simulink model "saturn_ib_stack_test"  (Simulink 6.2)
settings: Solver=ode4  SolverMode=SingleTasking  StartTime=-20.0  StopTime=620  FixedStep=0.005  RelTol=1e-3
values from neighbouring files (symbols this model uses):
  A_z_deg = 82.8200    (= 82.82)    [AS205_presettings.m]
  BN_1_sec = 14.4    [AS205_presettings.m]
  DeltaV_b_mps = 7.2381    [AS205_presettings.m]
  epsilon_2_sec = 15.0    (= 15)    [AS205_presettings.m]
  epsilon_prime_sec = 3.0    (= 3)    [AS205_presettings.m]
  i_deg = 28.89597    [AS205_presettings.m]
  lambda_0_deg = 102.32900    (= 102.329)    [AS205_presettings.m]
  lambda_L_deg = -80.561141    [AS205_presettings.m]
  pad_roll_L_deg = 100.0    (= 100)    [AS205_presettings.m]
  phi_L_deg = 28.521963    [AS205_presettings.m]
  phi_L_prime_deg = 28.360795    [AS205_presettings.m]
  R_L_m = 6373385.0    (= 6373385)    [AS205_presettings.m]
  R_T_m = 6570774.0    (= 6570774)    [AS205_presettings.m]
  T3_FM_sec = 6.08    [AS205_presettings.m]
  T_HSL_sec = 5.0    (= 5)    [AS205_presettings.m]
  Theta_T_deg = 0.000    (= 0)    [AS205_presettings.m]
  V_T_mps = 7780.976    [AS205_presettings.m]
  Xdotdot_VGT_mps2 = -9.251    [AS205_presettings.m]
undefined symbols (not defined in the file or in its folder): e0_0, e1_0, e2_0, e3_0, m, s
libraries: simulink x99, aerolibconvert x83, aerolibutil x63, aerolibtransform2 x34, aerolibasang x2, aerolibatmos2 x2, aerolib6dofsys x2
(part 1 of 7)
CloseFcn:
  | rtwprivate ssgencode ModelCloseRequest Saturn_IB_CSM_test
settings Model: LastModifiedBy=riley  StrictBusMsg=ErrorLevel1
settings OptimizationCC: InlineParams=on  InlineInvariantSignals=on  EnforceIntegerDowncast=off
settings DebuggingCC: ArrayBoundsChecking=error  SignalInfNanChecking=error  AlgebraicLoopMsg=error  SolverPrmCheckMsg=warning  IntegerOverflowMsg=error  SFcnCompatibilityMsg=error
settings RTWCC: SystemTargetFile=grt_malloc.tlc  GenCodeOnly=on  TemplateMakefile=grt_malloc_default_tmf  Description=Generic Real-Time Target with dynamic memory allocation  ProcessScript=grt_malloc_make_rtw_hook
settings GRTTargetCC: UtilityFuncGeneration=Shared location

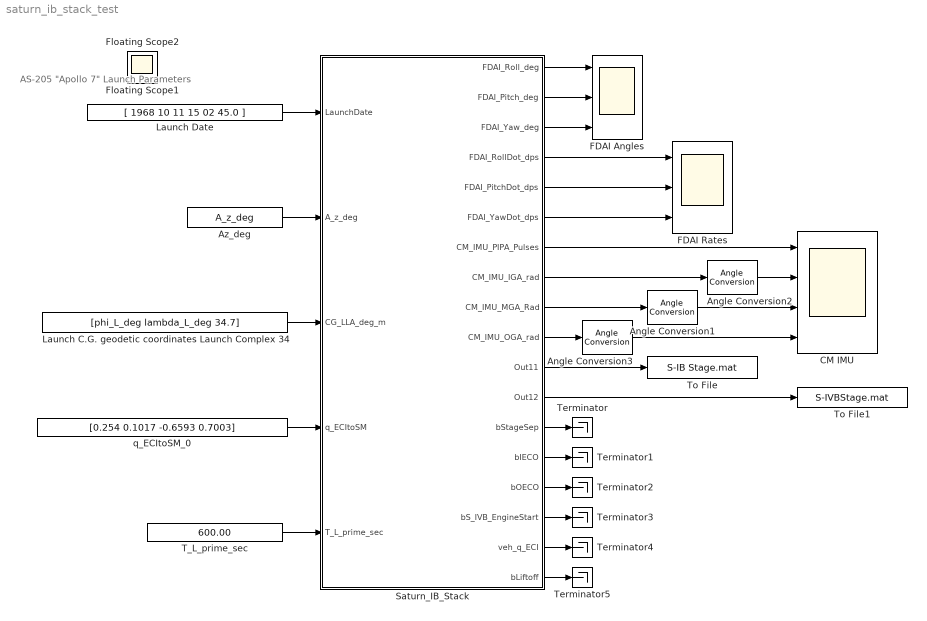
== system saturn_ib_stack_test ==
  note: AS-205 "Apollo 7" Launch Parameters
  Angle Conversion1 : aerolibconvert/Angle Conversion  IU=rad  OU=deg
  Angle Conversion2 : aerolibconvert/Angle Conversion  IU=rad  OU=deg
  Angle Conversion3 : aerolibconvert/Angle Conversion  IU=rad  OU=deg
  Az_deg : Constant  Value=A_z_deg
  CM IMU : Scope  NumInputPorts=4
      settings: YMin=-3500~90.002~-0.005~-17.188  YMax=500~90.015~0.035~-17.179  SaveName=ScopeData11
  FDAI Angles : Scope  NumInputPorts=3
      settings: YMin=-18~85.5~-0.02  YMax=0~90.25~0.06  SaveName=ScopeData8
  FDAI Rates : Scope  NumInputPorts=3
      settings: YMin=-0.07~-0.35~-0.05  YMax=0.005~-5.55112e-017~0.04  SaveName=ScopeData7
  Launch C.G. geodetic coordinates Launch Complex 34 : Constant  Value=[phi_L_deg lambda_L_deg 34.7]
  Launch Date : Constant  Value=[ 1968 10 11 15 02 45.0 ]
  Saturn_IB_Stack : Subsystem
  T_L_prime_sec : Constant  Value=600.00
  Terminator{,1..5} (6 alike) : Terminator
  To File : ToFile  Filename=S-IB Stage.mat  SampleTime=0.04
  To File1 : ToFile  Filename=S-IVBStage.mat  MatrixName=ans_sivb  SampleTime=0.04
  q_ECItoSM_0 : Constant  Value=[0.254 0.1017 -0.6593 0.7003]
  Floating Scope1 : Scope
      settings: Floating=on  SaveName=ScopeData16
  Floating Scope2 : Scope
      settings: Floating=on  SaveName=ScopeData17
  wires:
  Az_deg/1 -> Saturn_IB_Stack/2(A_z_deg)
  Launch Date/1 -> Saturn_IB_Stack/1(LaunchDate)
  Launch C.G. geodetic coordinates Launch Complex 34/1 -> Saturn_IB_Stack/3(CG_LLA_deg_m)
  Saturn_IB_Stack/4(FDAI_RollDot_dps) -> FDAI Rates/1
  Saturn_IB_Stack/7(CM_IMU_PIPA_Pulses) -> CM IMU/1
  Saturn_IB_Stack/10(CM_IMU_OGA_rad) -> Angle Conversion3/1
  Angle Conversion2/1 -> CM IMU/2
  Angle Conversion1/1 -> CM IMU/3
  Angle Conversion3/1 -> CM IMU/4
  Saturn_IB_Stack/1(FDAI_Roll_deg) -> FDAI Angles/1
  Saturn_IB_Stack/2(FDAI_Pitch_deg) -> FDAI Angles/2
  Saturn_IB_Stack/3(FDAI_Yaw_deg) -> FDAI Angles/3
  Saturn_IB_Stack/5(FDAI_PitchDot_dps) -> FDAI Rates/2
  Saturn_IB_Stack/6(FDAI_YawDot_dps) -> FDAI Rates/3
  Saturn_IB_Stack/8(CM_IMU_IGA_rad) -> Angle Conversion2/1
  Saturn_IB_Stack/9(CM_IMU_MGA_Rad) -> Angle Conversion1/1
  Saturn_IB_Stack/11(Out11) -> To File/1
  Saturn_IB_Stack/12(Out12) -> To File1/1
  Saturn_IB_Stack/13(bStageSep) -> Terminator/1
  Saturn_IB_Stack/14(bIECO) -> Terminator1/1
  Saturn_IB_Stack/15(bOECO) -> Terminator2/1
  Saturn_IB_Stack/16(bS_IVB_EngineStart) -> Terminator3/1
  q_ECItoSM_0/1 -> Saturn_IB_Stack/4(q_ECItoSM)
  Saturn_IB_Stack/17(veh_q_ECI) -> Terminator4/1
  Saturn_IB_Stack/18(bLiftoff) -> Terminator5/1
  T_L_prime_sec/1 -> Saturn_IB_Stack/5(T_L_prime_sec)

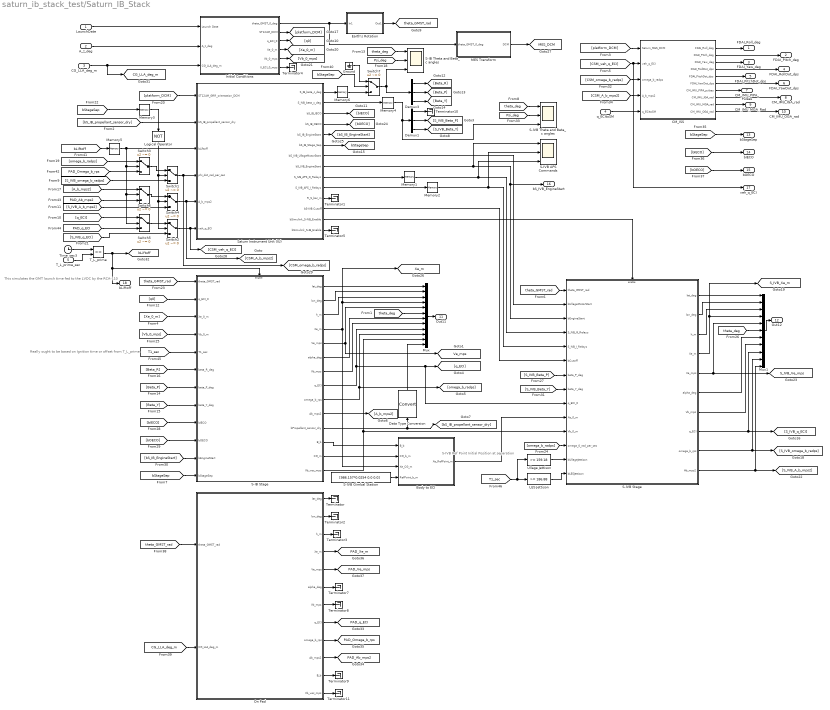
== system saturn_ib_stack_test/Saturn_IB_Stack ==
  note: S-IVB Ref Point Initial
      | Position at separation
  note: Really ought to be based on
      | Ignition time or offset
      | from T_L_prime
  note: This simulates the
      | GMT launch time
      | fed to the LVDC by
      | the RCA-110
  LaunchDate : Inport  Port=1  PortDimensions=6  DataType=double  LatchInput=off
  A_z_deg : Inport  Port=2  PortDimensions=1  DataType=double  LatchInput=off
  CG_LLA_deg_m : Inport  Port=3  PortDimensions=3  DataType=double  LatchInput=off
  q_ECItoSM : Inport  Port=4  PortDimensions=4  DataType=double  LatchInput=off
  T_L_prime_sec : Inport  Port=5  PortDimensions=1  DataType=double  LatchInput=off
  Body to ECI : Subsystem
  CM_ISS : Subsystem
  Data Type Conversion : DataTypeConversion  Orientation=up
  Demux1 : Demux  Outputs=3
  Demux3 : Demux  Outputs=3
  Earth's Rotation : Subsystem
  Ground : Ground
  Initial Conditions : Subsystem
  LES Jettison : simulink/Logic and Bit Operations/Compare To Constant  relop=>=  const=186.88  LogicOutDataTypeMode=boolean  ZeroCross=off
  Logical Operator : Logic  Orientation=down  Operator=NOT  AllPortsSameDT=off  OutDataTypeMode=Boolean
  MES Transform : Subsystem
  Memory{1..6} (6 alike) : Memory  InheritSampleTime=on
  Mux : Mux  Inputs=12
  Mux1 : Mux  Inputs=11
  On Pad : Subsystem
  S-IB Stage : Subsystem
  S-IB Theta and Beta_c angles : Scope  NumInputPorts=3
      settings: YMin=-18~-1.3~-0.04  YMax=1~0.3~0.14  SaveName=ScopeData2  Decimation=10  SampleTime=0.01
  S-IVB APS Commands : Scope  NumInputPorts=3
      settings: TimeRange=620  YMin=0.95~-1~-1  YMax=1.05~1~1  SaveName=ScopeData3  MaxDataPoints=15000  Decimation=10  SampleTime=0.01
  S-IVB Gimbal Station : Constant  Value=[986.157*0.0254 0.0 0.0]
  S-IVB Stage : Subsystem
  S-IVB Theta and Beta_c angles : Scope  NumInputPorts=3
      settings: YMin=-65~-0.075~-0.5  YMax=5~0.425~0.8  SaveName=ScopeData12  MaxDataPoints=15000  Decimation=10  SampleTime=0.01
  Saturn Instrument Unit (IU) : Subsystem
  Switch{1..7} (7 alike) : Switch  Criteria=u2 ~= 0
  T_L_prime : RelationalOperator  LogicOutDataTypeMode=Boolean
  Terminator{,1..5,7..11} (11 alike) : Terminator
  Time_sec3 : Clock
  Ullage Jettison : simulink/Logic and Bit Operations/Compare To Constant  relop=>=  const=159.18  LogicOutDataTypeMode=boolean  ZeroCross=off
  FDAI_Roll_deg : Outport  PortDimensions=1
  FDAI_Pitch_deg : Outport  Port=2  PortDimensions=1
  FDAI_Yaw_deg : Outport  Port=3  PortDimensions=1
  FDAI_RollDot_dps : Outport  Port=4
  FDAI_PitchDot_dps : Outport  Port=5
  FDAI_YawDot_dps : Outport  Port=6
  CM_IMU_PIPA_Pulses : Outport  Port=7
  CM_IMU_IGA_rad : Outport  Port=8
  CM_IMU_MGA_Rad : Outport  Port=9
  CM_IMU_OGA_rad : Outport  Port=10
  Out11 : Outport  Port=11
  Out12 : Outport  Port=12
  bStageSep : Outport  Port=13  DataType=boolean
  bIECO : Outport  Port=14  DataType=boolean
  bOECO : Outport  Port=15  DataType=boolean
  bS_IVB_EngineStart : Outport  Port=16  DataType=boolean
  veh_q_ECI : Outport  Port=17  PortDimensions=4  DataType=double
  bLiftoff : Outport  Port=18  DataType=boolean
  tag scope: CG_LLA_deg_m=global, MES_DCM=global, PAD_Ab_mps2=global, PAD_Omega_b_rps=global, PAD_Ve_mps=global, PAD_Xe_m=global, PAD_q_ECI=global, S_IVB_Ve_mps=global, S_IVB_Xe_m=global, Ve_mps=global, Xe_m=global, bLiftoff=global, bStageSep=global, theta_GMST_rad=global
  wires:
  Earth's Rotation/1(Out1) -> [theta_GMST_rad]
  Initial Conditions/1(theta_GMST_0_deg) -> Earth's Rotation/1(In1), MES Transform/1(theta_GMST_0_deg)
  Initial Conditions/3(q_ECI_0) -> [q0]
  Initial Conditions/2(ST124M_DCM) -> [platform_DCM]
  [q0] -> S-IB Stage/2(q_ECI_0)
  [theta_GMST_rad] -> S-IB Stage/1(theta_GMST_rad)
  Initial Conditions/4(Xe_0_m) -> [Xe_0_m]
  [Xe_0_m] -> S-IB Stage/3(Xe_0_m)
  [Beta_Y] -> S-IB Stage/8(beta_Y_deg)
  Initial Conditions/5(Vb_0_mps) -> [Vb_0_mps]
  [Vb_0_mps] -> S-IB Stage/4(Vb_0_m)
  [Beta_R] -> S-IB Stage/6(beta_R_deg)
  [Beta_P] -> S-IB Stage/7(beta_P_deg)
  Demux3/3 -> [Beta_Y]
  Demux3/1 -> [Beta_R]
  Demux3/2 -> [Beta_P]
  [Psi_deg] -> S-IB Theta and Beta_c angles/2
  [theta_deg] -> S-IB Theta and Beta_c angles/1
  [platform_DCM] -> Saturn Instrument Unit (IU)/1(ST124M_GRR_orientation_DCM)
  [bS_IB_EngineStart] -> S-IB Stage/11(bEngineStart)
  [bOECO] -> S-IB Stage/10(bOECO)
  [bIECO] -> S-IB Stage/9(bIECO)
  S-IB Stage/4(Xe_m) -> Body to ECI/3(Xe_CG_m), Mux/4, [Xe_m]
  S-IB Stage/5(Ve_mps) -> [Ve_mps], Mux/5
  Saturn Instrument Unit (IU)/3(bS_IB_IECO) -> [bIECO]
  Saturn Instrument Unit (IU)/4(bS_IB_OECO) -> [bOECO]
  Saturn Instrument Unit (IU)/5(bS_IB_EngineStart) -> [bS_IB_EngineStart]
  S-IB Stage/1(lat_deg) -> Mux/1
  S-IB Stage/2(lon_deg) -> Mux/2
  S-IB Stage/3(h_m) -> Mux/3
  S-IB Stage/6(alpha_deg) -> Mux/7
  S-IB Stage/7(Vb_mps) -> Mux/8
  [theta_deg] -> Mux/6
  S-IB Stage/8(q_ECI) -> Mux/9, [q_ECI], S-IVB Stage/9(q_ECI_0)
  S-IB Stage/9(omega_b_rps) -> [omega_b_radps], Mux/10
  S-IB Stage/10(Ab_mps2) -> [A_b_mps2]
  [bS_IB_propellant_sensor_dry] -> Saturn Instrument Unit (IU)/2(bS_IB_propellant_sensor_dry)
  S-IB Stage/12(B_b) -> Body to ECI/1(B_b)
  S-IB Stage/13(CG_m) -> Body to ECI/2(CG_b_m)
  S-IVB Gimbal Station/1 -> Body to ECI/4(RefPoint_b_m)
  [bStageSep] -> S-IB Stage/12(bStageSep)
  Demux1/3 -> [S_IVB_Beta_Y]
  Demux1/1 -> Terminator10/1
  Demux1/2 -> [S_IVB_Beta_P]
  Saturn Instrument Unit (IU)/2(S_IVB_beta_c_deg) -> Memory4/1
  Switch2/1 -> Saturn Instrument Unit (IU)/6(veh_q_ECI), [CSM_veh_q_ECI]
  [S_IVB_omega_b_radps] -> Switch1/3
  [S_IVB_A_b_mps2] -> Switch4/3
  [S_IVB_q_ECI] -> Switch2/3
  [bStageSep] -> Memory3/1
  Logical Operator/1 -> Switch2/2, Switch4/2, Switch1/2
  S-IB Stage/14(Vb_vec_mps) -> Mux/11, S-IVB Stage/11(Vb_0_m)
  Data Type Conversion/1 -> Mux/12
  Initial Conditions/6(V_ECI_0_mps) -> Terminator4/1
  Saturn Instrument Unit (IU)/7(bS_IVB_UllageMotorStart) -> S-IVB Stage/2(bUllageMotorStart)
  Saturn Instrument Unit (IU)/8(bS_IVB_EngineStart) -> S-IVB APS Commands/1, S-IVB Stage/3(bEngineStart), bS_IVB_EngineStart/1
  Saturn Instrument Unit (IU)/9(S_IVB_APS_III_Relays) -> Memory1/1
  Saturn Instrument Unit (IU)/10(S_IVB_APS_I_Relays) -> Memory2/1
  Saturn Instrument Unit (IU)/13(bSimulink_S-IVB_Enable) -> S-IVB Stage/Enable
  S-IB Stage/11(bPropellant_sensor_dry) -> [bS_IB_propellant_sensor_dry], Data Type Conversion/1
  Saturn Instrument Unit (IU)/14(bSimulink_S-IB_Enable) -> Terminator5/1
  Switch1/1 -> [CSM_omega_b_radps], Saturn Instrument Unit (IU)/4(phi_dot_rad_per_sec)
  Switch4/1 -> Saturn Instrument Unit (IU)/5(A_b_mps2), [CSM_A_b_mps2]
  Saturn Instrument Unit (IU)/6(bS_IB_Stage_Sep) -> [bStageSep]
  S-IVB Stage/1(lat_deg) -> Mux1/1
  S-IVB Stage/6(alpha_deg) -> Mux1/7
  S-IVB Stage/5(Ve_mps) -> [S_IVB_Ve_mps], Mux1/5
  S-IVB Stage/2(lon_deg) -> Mux1/2
  [theta_GMST_rad] -> S-IVB Stage/1(theta_GMST_rad)
  Saturn Instrument Unit (IU)/12(bS-IVB Cutoff) -> S-IVB Stage/6(bCutoff)
  [S_IVB_Beta_P] -> S-IVB Stage/7(beta_P_deg)
  [S_IVB_Beta_Y] -> S-IVB Stage/8(beta_Y_deg)
  Body to ECI/1(Xe_RefPoint_m) -> S-IVB Stage/10(Xe_0_m)
  S-IVB Stage/8(q_ECI) -> [S_IVB_q_ECI], Mux1/9
  S-IVB Stage/9(omega_b_rps) -> [S_IVB_omega_b_radps], Mux1/10
  S-IVB Stage/10(Ab_mps2) -> [S_IVB_A_b_mps2], Mux1/11
  S-IVB Stage/7(Vb_mps) -> Mux1/8
  [theta_deg] -> Mux1/6
  S-IVB Stage/3(h_m) -> Mux1/3
  S-IVB Stage/4(Xe_m) -> Mux1/4, [S_IVB_Xe_m]
  [omega_b_radps] -> S-IVB Stage/12(omega_0_rad_per_sec)
  Memory1/1 -> S-IVB Stage/4(S_IVB_III_Relays), S-IVB APS Commands/3
  Memory3/1 -> Logical Operator/1
  [theta_deg] -> S-IVB Theta and Beta_c angles/1
  [Psi_deg] -> S-IVB Theta and Beta_c angles/2
  Ullage Jettison/1 -> S-IVB Stage/13(bUllageJettison)
  LES Jettison/1 -> S-IVB Stage/14(bLESJettison)
  MES Transform/1(DCM) -> [MES_DCM]
  Memory2/1 -> S-IVB Stage/5(S_IVB_I_Relays), S-IVB APS Commands/2
  Memory4/1 -> Demux1/1, S-IVB Theta and Beta_c angles/3
  Saturn Instrument Unit (IU)/11(R_S_bar_m) -> Terminator1/1
  [platform_DCM] -> CM_ISS/1(Saturn_MES_DCM)
  [CSM_veh_q_ECI] -> CM_ISS/2(veh_q_ECI), veh_q_ECI/1
  [CSM_omega_b_radps] -> CM_ISS/3(omega_b_radps)
  [CSM_A_b_mps2] -> CM_ISS/4(A_b_mps2)
  LaunchDate/1 -> Initial Conditions/1(Launch Date)
  A_z_deg/1 -> Initial Conditions/2(A_z_deg)
  CM_ISS/1(FDAI_Roll_deg) -> FDAI_Roll_deg/1
  CM_ISS/2(FDAI_Pitch_deg) -> FDAI_Pitch_deg/1
  CM_ISS/3(FDAI_Yaw_deg) -> FDAI_Yaw_deg/1
  CG_LLA_deg_m/1 -> Initial Conditions/3(CG_LLA_deg_m), [CG_LLA_deg_m]
  CM_ISS/4(FDAI_RollDot_dps) -> FDAI_RollDot_dps/1
  CM_ISS/5(FDAI_PitchDot_dps) -> FDAI_PitchDot_dps/1
  CM_ISS/6(FDAI_YawDot_dps) -> FDAI_YawDot_dps/1
  CM_ISS/7(CM_IMU_PIPA_pulses) -> CM_IMU_PIPA_Pulses/1
  CM_ISS/8(CM_IMU_IGA_rad) -> CM_IMU_IGA_rad/1
  CM_ISS/9(CM_IMU_MGA_rad) -> CM_IMU_MGA_Rad/1
  CM_ISS/10(CM_IMU_OGA_rad) -> CM_IMU_OGA_rad/1
  Mux/1 -> Out11/1
  Mux1/1 -> Out12/1
  [bStageSep] -> bStageSep/1
  [bIECO] -> bIECO/1
  [bOECO] -> bOECO/1
  q_ECItoSM/1 -> CM_ISS/5(q_ECItoSM)
  [theta_GMST_rad] -> On Pad/1(theta_GMST_rad)
  [CG_LLA_deg_m] -> On Pad/2(CG_LLA_deg_m)
  T_L_prime/1 -> [bLiftoff], S-IB Stage/Enable, bLiftoff/1
  On Pad/8(q_ECI) -> [PAD_q_ECI]
  On Pad/10(Ab_mps2) -> [PAD_Ab_mps2]
  On Pad/9(omega_b_rps) -> [PAD_Omega_b_rps]
  On Pad/1(lat_deg) -> Terminator/1
  On Pad/2(lon_deg) -> Terminator2/1
  On Pad/3(h_m) -> Terminator3/1
  On Pad/4(Xe_m) -> [PAD_Xe_m]
  On Pad/5(Ve_mps) -> [PAD_Ve_mps]
  On Pad/6(alpha_deg) -> Terminator7/1
  On Pad/7(Vb_mps) -> Terminator8/1
  On Pad/11(B_b) -> Terminator9/1
  On Pad/12(Vb_vec_mps) -> Terminator11/1
  Switch3/1 -> Switch1/1
  [omega_b_radps] -> Switch3/1
  Switch6/1 -> Switch4/1
  Switch5/1 -> Switch2/1
  [A_b_mps2] -> Switch6/1
  [q_ECI] -> Switch5/1
  [bLiftoff] -> Memory5/1
  [PAD_Omega_b_rps] -> Switch3/3
  [PAD_q_ECI] -> Switch5/3
  [PAD_Ab_mps2] -> Switch6/3
  Memory5/1 -> Switch3/2, Switch6/2, Switch5/2, Saturn Instrument Unit (IU)/3(bLiftoff)
  Saturn Instrument Unit (IU)/1(S_IB_beta_c_deg) -> Memory6/1
  Switch7/1 -> Demux3/1, S-IB Theta and Beta_c angles/3
  [bStageSep] -> Switch7/2
  Ground/1 -> Switch7/1
  Memory6/1 -> Switch7/3
  [T1_sec] -> S-IB Stage/5(T1_sec)
  Time_sec3/1 -> T_L_prime/1
  T_L_prime_sec/1 -> T_L_prime/2
  [T1_sec] -> LES Jettison/1, Ullage Jettison/1

== system saturn_ib_stack_test/Saturn_IB_Stack/Body to ECI ==
  note: ECI to Body Transform
  note: Convert a point in Body coordinates
      | io ECI coordinates.
  note: Point (body frame)
  note: C.G. (body Frame)
  note: C.G. Location (ECI Frame)
  B_b : Inport  Port=1  PortDimensions=[3 3]  LatchInput=off
  CG_b_m : Inport  Port=2  PortDimensions=3  LatchInput=off
  Xe_CG_m : Inport  Port=3  PortDimensions=3  LatchInput=off
  RefPoint_b_m : Inport  Port=4  PortDimensions=3  LatchInput=off
  Math Function : Math  Operator=transpose  SaturateOnIntegerOverflow=on
  Product : Product  Multiplication=Matrix(*)  RndMeth=Zero
  Sum : Sum  Inputs=|++
  Sum1 : Sum  Inputs=|+-
  Xe_RefPoint_m : Outport
  wires:
  B_b/1 -> Math Function/1
  Math Function/1 -> Product/1
  Sum/1 -> Xe_RefPoint_m/1
  Xe_CG_m/1 -> Sum/2
  Sum1/1 -> Product/2
  RefPoint_b_m/1 -> Sum1/1
  CG_b_m/1 -> Sum1/2
  Product/1 -> Sum/1

== system saturn_ib_stack_test/Saturn_IB_Stack/CM_ISS ==
  note: Direction cosine matrix, X_S is down,
      | Z_S points downrange
  note: Simulate PIPA Pulse counters
      | which are acceeration integrators.
      | These values include accelerations
      | sensed due to gravity.
  note: Output the total pulse count
      | (as a whole number) -- external code
      | must look for changes at each time step
      | and update the AGC counters as required.
  Saturn_MES_DCM : Inport  Port=1  LatchInput=off
  veh_q_ECI : Inport  Port=2  PortDimensions=4  DataType=double  LatchInput=off
  omega_b_radps : Inport  Port=3  LatchInput=off
  A_b_mps2 : Inport  Port=4  PortDimensions=3  LatchInput=off
  q_ECItoSM : Inport  Port=5  LatchInput=off
  Angle Conversion{,1..3} (4 alike) : aerolibconvert/Angle Conversion  IU=rad  OU=deg
  BODYtoECI : Math  Operator=transpose  SaturateOnIntegerOverflow=on
  Demux : Demux  Outputs=3
  Demux2 : Demux  Outputs=3
  Demux3 : Demux  Outputs=3
  ECItoBODY : aerolibtransform2/Quaternions to  Direction Cosine Matrix
  ECItoSM : aerolibtransform2/Quaternions to  Direction Cosine Matrix
  M2SM : Constant  Value=[ 0.0 0.0 1.0; 0.0 1.0 0.0; -1.0 0.0 0.0]
  M2SM1 : Constant  Value=[ 0.0 0.0 1.0; 0.0 1.0 0.0; -1.0 0.0 0.0]
  Math Function : Math  Operator=transpose  SaturateOnIntegerOverflow=on
  Math Function2 : Math  Operator=transpose  SaturateOnIntegerOverflow=on
  Mux : Mux  Inputs=3
  Product{1..4,9} (5 alike) : Product  Multiplication=Matrix(*)  RndMeth=Zero
  Quaternions to  Direction Cosine Matrix1 : aerolibtransform2/Quaternions to  Direction Cosine Matrix
  Rounding Function : Rounding
  Rounding Function1 : Rounding
  Rounding Function2 : Rounding
  Stable Member Gimbal Angles : Subsystem  AncestorBlock=aerolibtransform2/Direction Cosine Matrix to Euler Angles
      mask Type: DCM2Euler
      mask Description: Determine equivalent ST-124M Gimbal angles from the 3-by-3 direction cosine matrix (DCM). The input DCM transforms vectors from Body frame to S-Frame.  EDD Equation 2.3.3 was used to determine the correct Euler angle rotation sequence used in the ST-124M.
      mask Display: disp('SM2Gimbal')
  Stable Member Gimbal Angles1 : Subsystem  AncestorBlock=aerolibtransform2/Direction Cosine Matrix to Euler Angles
      mask Type: DCM2Euler
      mask Description: Determine equivalent ST-124M Gimbal angles from the 3-by-3 direction cosine matrix (DCM). The input DCM transforms vectors from Body frame to S-Frame.  EDD Equation 2.3.3 was used to determine the correct Euler angle rotation sequence used in the ST-124M.
      mask Display: disp('SM2Gimbal')
  Terminator : Terminator
  m/sec to pulses : Gain  Gain=100.0/5.85
  velocity in SM frame : Integrator
  FDAI_Roll_deg : Outport
  FDAI_Pitch_deg : Outport  Port=2
  FDAI_Yaw_deg : Outport  Port=3
  FDAI_RollDot_dps : Outport  Port=4
  FDAI_PitchDot_dps : Outport  Port=5
  FDAI_YawDot_dps : Outport  Port=6
  CM_IMU_PIPA_pulses : Outport  Port=7  PortDimensions=3  DataType=double
  CM_IMU_IGA_rad : Outport  Port=8  PortDimensions=1  DataType=double
  CM_IMU_MGA_rad : Outport  Port=9  PortDimensions=1  DataType=double
  CM_IMU_OGA_rad : Outport  Port=10  PortDimensions=1  DataType=double
  wires:
  Product9/1 -> Math Function2/1
  Quaternions to  Direction Cosine Matrix1/1 -> Product9/1
  Math Function/1 -> Product9/2
  veh_q_ECI/1 -> Quaternions to  Direction Cosine Matrix1/1, ECItoBODY/1
  Math Function2/1 -> Product1/2
  Product1/1 -> Stable Member Gimbal Angles/1(DCM)
  M2SM/1 -> Product1/1
  Saturn_MES_DCM/1 -> Math Function/1
  omega_b_radps/1 -> Angle Conversion/1
  Angle Conversion/1 -> Demux/1
  Demux/1 -> FDAI_RollDot_dps/1
  Demux/2 -> FDAI_PitchDot_dps/1
  Demux/3 -> FDAI_YawDot_dps/1
  Stable Member Gimbal Angles/1(CM IMU Gimbal) -> Terminator/1
  velocity in SM frame/1 -> m/sec to pulses/1
  Mux/1 -> CM_IMU_PIPA_pulses/1
  Product2/1 -> velocity in SM frame/1
  A_b_mps2/1 -> Product2/2
  m/sec to pulses/1 -> Demux2/1
  Demux2/1 -> Rounding Function/1
  Demux2/2 -> Rounding Function1/1
  Demux2/3 -> Rounding Function2/1
  Rounding Function/1 -> Mux/1
  Rounding Function1/1 -> Mux/2
  Rounding Function2/1 -> Mux/3
  Angle Conversion3/1 -> FDAI_Pitch_deg/1
  Angle Conversion1/1 -> FDAI_Yaw_deg/1
  Angle Conversion2/1 -> FDAI_Roll_deg/1
  ECItoBODY/1 -> BODYtoECI/1
  q_ECItoSM/1 -> ECItoSM/1
  Stable Member Gimbal Angles1/1(CM IMU Gimbal) -> Demux3/1
  Demux3/1 -> Angle Conversion3/1, CM_IMU_IGA_rad/1
  Demux3/2 -> Angle Conversion1/1, CM_IMU_MGA_rad/1
  Demux3/3 -> Angle Conversion2/1, CM_IMU_OGA_rad/1
  ECItoSM/1 -> Product3/1
  BODYtoECI/1 -> Product3/2
  Product4/1 -> Stable Member Gimbal Angles1/1(DCM), Product2/1
  Product3/1 -> Product4/2
  M2SM1/1 -> Product4/1

== system saturn_ib_stack_test/Saturn_IB_Stack/Earth's Rotation ==
  In1 : Inport  Port=1  LatchInput=off
  Angle Conversion3 : aerolibconvert/Angle Conversion  IU=deg  OU=rad
  Product2 : Product  RndMeth=Zero
  Sum : Sum  Inputs=|++
  Time_sec : Clock
  omega_e_rad_per_sec : Constant  Value=7.292115e-05
  Out1 : Outport
  wires:
  Product2/1 -> Sum/2
  Angle Conversion3/1 -> Sum/1
  omega_e_rad_per_sec/1 -> Product2/1
  Time_sec/1 -> Product2/2
  In1/1 -> Angle Conversion3/1
  Sum/1 -> Out1/1

== system saturn_ib_stack_test/Saturn_IB_Stack/Initial Conditions ==
  note: Compare MES-based calculations
      | from EDD to my DIS-based computation
  Launch Date : Inport  Port=1  LatchInput=off
  A_z_deg : Inport  Port=2  LatchInput=off
  CG_LLA_deg_m : Inport  Port=3  LatchInput=off
  3x3 Cross Product : aerolibutil/3x3 Cross Product
  Angle Conversion : aerolibconvert/Angle Conversion  IU=deg  OU=rad
  Angle Conversion1 : aerolibconvert/Angle Conversion  IU=deg  OU=rad
  Angle Conversion2 : aerolibconvert/Angle Conversion  IU=deg  OU=rad
  Date to JD : Subsystem
  Demux : Demux  Outputs=3
  Direction Cosine Matrix  to Quaternion : aerolibtransform2/Direction Cosine Matrix  to Quaternions
  Euler Angles to  Direction Cosine Matrix : aerolibtransform2/Euler Angles to  Direction Cosine Matrix
  Initial Position and Velocity (Eqns. 3.4.3-4) : Subsystem  mask{omega_E_rps=0.000023211523}
  L/V Inertial Orientation : Subsystem  TreatAsAtomicUnit=on  SystemSampleTime=0.8
  LLA to ECF : Subsystem
  MES Transform : Subsystem
  Math Function : Math  Operator=transpose  SaturateOnIntegerOverflow=on
  Mux : Mux  Inputs=3
  Position 1  Azimuth (deg) : Constant  Value=pad_roll_L_deg
  Product{,1..3} (4 alike) : Product  Multiplication=Matrix(*)  RndMeth=Zero
  R_L : Constant  Value=R_L_m
  Reshape 9x1 : simulink/Math Operations/Reshape  OutputDimensionality=Row vector  OutputDimensions=[3,3]
  Reshape 9x2 : simulink/Math Operations/Reshape  OutputDimensionality=Row vector  OutputDimensions=[3,3]
  Sum : Sum  Inputs=|++
  Sum1 : Sum  Inputs=+-|
  Sum2 : Sum  Inputs=+-|
  T to GMST : Subsystem
  T_UT1 : Fcn  Expr=(u(1) - 2451545.0) / 36525
  To File : ToFile  Filename=saturn-MES-frame.mat  MatrixName=MES
      settings: Decimation=1000
  To File1 : ToFile  Filename=saturn-Launch-frame.mat  MatrixName=MEL
      settings: Decimation=1000
  To Workspace : ToWorkspace  VariableName=Xe_error_m  SampleTime=-1  SaveFormat=Structure
      settings: Decimation=10000
  To Workspace1 : ToWorkspace  VariableName=Ve_error_mps  SampleTime=-1  SaveFormat=Structure
      settings: Decimation=10000
  Unary Minus : simulink/Math Operations/Unary Minus  DoSatur=off
  omega_E_rad_per_sec : Constant  Value=[0.0 0.0 7.292115E-05]
  phi_L_prime_deg : Constant  Value=phi_L_prime_deg
  zero : Constant  Value=0
  theta_GMST_0_deg : Outport
  ST124M_DCM : Outport  Port=2
  q_ECI_0 : Outport  Port=3
  Xe_0_m : Outport  Port=4
  Vb_0_mps : Outport  Port=5
  V_ECI_0_mps : Outport  Port=6
  wires:
  Date to JD/1(JD) -> T_UT1/1
  Launch Date/1 -> Date to JD/1(Date  (YYYY,mm,dd,hh,mm,ss.s))
  T_UT1/1 -> T to GMST/1(T_UT1)
  A_z_deg/1 -> Initial Position and Velocity (Eqns. 3.4.3-4)/2(A_z_deg)
  Direction Cosine Matrix  to Quaternion/1 -> q_ECI_0/1
  Demux/1 -> Angle Conversion/1, Initial Position and Velocity (Eqns. 3.4.3-4)/3(phi_L_deg), L/V Inertial Orientation/2(phi_L_deg)  "phi_L_deg"
  Demux/2 -> Angle Conversion1/1, Sum/2  "lambda_L_deg"
  Angle Conversion/1 -> LLA to ECF/1(lat (rad))
  Angle Conversion1/1 -> LLA to ECF/2(lon (rad))
  Demux/3 -> LLA to ECF/3(h (m))
  CG_LLA_deg_m/1 -> Demux/1
  LLA to ECF/1(XYZ (m)) -> Product/2
  Product/1 -> Xe_0_m/1, 3x3 Cross Product/2, Sum1/1
  Euler Angles to  Direction Cosine Matrix/1 -> Product/1
  Mux/1 -> Euler Angles to  Direction Cosine Matrix/1
  zero/1 -> Mux/1, Mux/2
  Angle Conversion2/1 -> Mux/3
  [A] -> Unary Minus/1
  omega_E_rad_per_sec/1 -> 3x3 Cross Product/1
  Product1/1 -> Vb_0_mps/1
  3x3 Cross Product/1 -> Product1/2, V_ECI_0_mps/1, Sum2/1  "V_ECI_0_mps"
  [A] -> Sum/1, MES Transform/1(theta_GMST_0_deg)
  Sum/1 -> L/V Inertial Orientation/3(Theta_E_deg)
  L/V Inertial Orientation/1(DCM) -> Direction Cosine Matrix  to Quaternion/1, Product1/1, Reshape 9x2/1
  Position 1  Azimuth (deg)/1 -> L/V Inertial Orientation/1(A_z_deg)
  Unary Minus/1 -> Angle Conversion2/1
  T to GMST/1(theta_GMST) -> theta_GMST_0_deg/1, [A]
  MES Transform/1(DCM) -> Reshape 9x1/1, ST124M_DCM/1, [MES]
  Reshape 9x1/1 -> To File/1
  Reshape 9x2/1 -> To File1/1
  R_L/1 -> Initial Position and Velocity (Eqns. 3.4.3-4)/1(R_L_m)
  phi_L_prime_deg/1 -> Initial Position and Velocity (Eqns. 3.4.3-4)/4(phi_L_prime_deg)
  [MES] -> Math Function/1
  Math Function/1 -> Product2/1, Product3/1
  Initial Position and Velocity (Eqns. 3.4.3-4)/1(R_S_0_m) -> Product2/2
  Initial Position and Velocity (Eqns. 3.4.3-4)/2(V_S_0_mps) -> Product3/2
  Product2/1 -> Sum1/2
  Product3/1 -> Sum2/2
  Sum1/1 -> To Workspace/1
  Sum2/1 -> To Workspace1/1

== system saturn_ib_stack_test/Saturn_IB_Stack/MES Transform ==
  theta_GMST_0_deg : Inport  Port=1  LatchInput=off
  Constant2 : Constant  Value=A_z_deg
  Constant8 : Constant  Value=phi_L_deg
  Constant9 : Constant  Value=lambda_L_deg
  MES Transform : Subsystem  TreatAsAtomicUnit=on  SystemSampleTime=0.8
  Sum2 : Sum  Inputs=|++
  DCM : Outport
  wires:
  Constant2/1 -> MES Transform/1(A_z_deg)
  Constant8/1 -> MES Transform/2(phi_L_deg)
  Constant9/1 -> Sum2/1
  Sum2/1 -> MES Transform/3(Theta_E_deg)
  theta_GMST_0_deg/1 -> Sum2/2
  MES Transform/1(DCM) -> DCM/1

== system saturn_ib_stack_test/Saturn_IB_Stack/On Pad ==
  note: Accelerometer sensor inputs
  note: Body-frame acceleration
      | due to gravity
  note: ECI to Body Transform
  note: Track state of the launch vechicle
      | while on the pad
  theta_GMST_rad : Inport  Port=1  LatchInput=off
  CG_LLA_deg_m : Inport  Port=2  LatchInput=off
  Add2 : Sum  Inputs=--  OutScaling=2^-10
  Angle Conversion4 : aerolibconvert/Angle Conversion  IU=rad  OU=deg
  Angle Conversion5 : aerolibconvert/Angle Conversion  IU=rad  OU=deg
  Centrifugal Acceleration : Subsystem
  Display13 : Display
  Display15 : Display
  ECI to LLA : Subsystem
  Earth Gravity Model : Subsystem
  Ground : Ground
  Initial Conditions : Subsystem
  Product : Product  Multiplication=Matrix(*)  RndMeth=Zero
  Product1 : Product  Multiplication=Matrix(*)  RndMeth=Zero
  Quaternions to  Direction Cosine Matrix : aerolibtransform2/Quaternions to  Direction Cosine Matrix
  Terminator : Terminator
  Terminator1 : Terminator
  height (m) : Display
  omega_E_rad_per_sec : Constant  Value=[0.0 0.0 7.292115E-05]
  lat_deg : Outport
  lon_deg : Outport  Port=2
  h_m : Outport  Port=3
  Xe_m : Outport  Port=4
  Ve_mps : Outport  Port=5
  alpha_deg : Outport  Port=6
  Vb_mps : Outport  Port=7
  q_ECI : Outport  Port=8
  omega_b_rps : Outport  Port=9  InitialOutput=[0.0 0.0 0.0]
  Ab_mps2 : Outport  Port=10  InitialOutput=[0.0 0.0 0.0]
  B_b : Outport  Port=11
  Vb_vec_mps : Outport  Port=12
  wires:
  ECI to LLA/3(h_ellp_m) -> h_m/1, height (m)/1
  [B_b] -> Product/1
  Earth Gravity Model/1(g (m/s^2)) -> Product/2
  Product/1 -> [g_b_mps2]
  [Xe_m] -> Earth Gravity Model/1(ECI_pos (m))
  Product1/1 -> omega_b_rps/1
  Initial Conditions/3(q_ECI) -> q_ECI/1, Quaternions to  Direction Cosine Matrix/1
  Angle Conversion4/1 -> lon_deg/1, Display13/1
  ECI to LLA/2(Lon_rad) -> Angle Conversion4/1
  ECI to LLA/1(Lat_rad) -> Angle Conversion5/1
  Angle Conversion5/1 -> Display15/1, lat_deg/1
  Initial Conditions/5(Vb_mps) -> Vb_vec_mps/1
  Add2/1 -> Ab_mps2/1
  [g_b_mps2] -> Add2/2
  theta_GMST_rad/1 -> Earth Gravity Model/2(theta_GMST_rad), ECI to LLA/1(theta_GMST_rad), Initial Conditions/1(Theta_GMST_rad)
  CG_LLA_deg_m/1 -> Initial Conditions/2(CG_LLA_deg_m)
  Quaternions to  Direction Cosine Matrix/1 -> B_b/1, Centrifugal Acceleration/2(ECItoBody), [B_b]
  Initial Conditions/4(Xe_m) -> Xe_m/1, ECI to LLA/2(ECI_pos (m)), [Xe_m], Centrifugal Acceleration/1(Xe_m)
  Initial Conditions/6(V_ECI_mps) -> Ve_mps/1
  Ground/1 -> Vb_mps/1, alpha_deg/1
  Centrifugal Acceleration/1(Out1) -> Add2/1
  Initial Conditions/1(theta_GMST_deg) -> Terminator/1
  Initial Conditions/2(ST124M_DCM) -> Terminator1/1
  [B_b] -> Product1/1
  omega_E_rad_per_sec/1 -> Product1/2

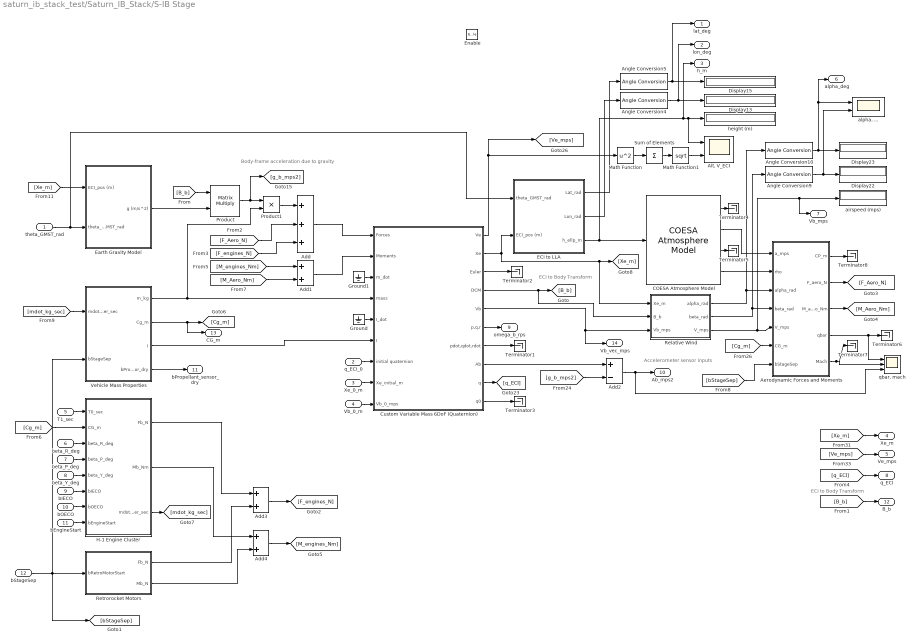
== system saturn_ib_stack_test/Saturn_IB_Stack/S-IB Stage ==
  note: Accelerometer sensor inputs
  note: Body-frame acceleration
      | due to gravity
  note: ECI to Body Transform
  note: ECI to Body Transform
  theta_GMST_rad : Inport  Port=1  LatchInput=off
  q_ECI_0 : Inport  Port=2  LatchInput=off
  Xe_0_m : Inport  Port=3  LatchInput=off
  Vb_0_m : Inport  Port=4  LatchInput=off
  T1_sec : Inport  Port=5  LatchInput=off
  beta_R_deg : Inport  Port=6  LatchInput=off
  beta_P_deg : Inport  Port=7  LatchInput=off
  beta_Y_deg : Inport  Port=8  LatchInput=off
  bIECO : Inport  Port=9  LatchInput=off
  bOECO : Inport  Port=10  LatchInput=off
  bEngineStart : Inport  Port=11  LatchInput=off
  bStageSep : Inport  Port=12  LatchInput=off
  Enable : EnablePort  StatesWhenEnabling=reset
  Add : Sum  Inputs=+++  OutScaling=2^-10
  Add1 : Sum  OutScaling=2^-10
  Add2 : Sum  Inputs=+-  OutScaling=2^-10
  Add3 : Sum  OutScaling=2^-10
  Add4 : Sum  OutScaling=2^-10
  Aerodynamic Forces and Moments : Subsystem
  "Alt, V_ECI" : Scope  NumInputPorts=2
      settings: TimeRange=140  YMin=5200~523.5  YMax=5400~526.25  Decimation=10
  Angle Conversion{4..5,9..10} (4 alike) : aerolibconvert/Angle Conversion  IU=rad  OU=deg
  COESA Atmosphere Model : aerolibatmos2/COESA Atmosphere Model  units=Metric (MKS)  spec=1976 COESA-extended U.S. Standard Atmosphere  model=Profile  profile_var=High temperature  profile_percent=1%  profile_alt=5 km (16404 ft)  envelope_var=High temperature  envelope_percent=1%  action=Warning
  Custom Variable Mass 6DoF (Quaternion) : Subsystem  mask(6DoF EoM (Body Axis)){units=Metric (MKS), mtype=Custom Variable, rep=Quaternion, xme_0=[0 0 0], Vm_0=[0 0 0], eul_0=[0 0 0], pm_0=[0 0 0], mass_0=1.0, mass_e=0, mass_f=0, inertia=eye(3), inertia_e=eye(3), inertia_f=eye(3), k_quat=1.0}
      mask prompts: mtype "Mass type:"; rep "Representation:"; xme_0 "Initial position in inertial axes [Xe,Ye,Ze]:"; Vm_0 "Initial velocity in body axes [U,v,w]:"; eul_0 "Initial Euler orientation [roll, pitch, yaw]:"; pm_0 "Initial body rotation rates [p,q,r]:"; mass_0 "Initial mass:"; mass_e "Empty mass:"; mass_f "Full mass:"; inertia_e "Empty inertia matrix:"; inertia_f "Full inertia matrix:"; k_quat "Gain for quaternion normalization:"
      mask help: Integrate the six-degrees-of-freedom equations of motion using an Euler angle representation for the orientation of the body in space.
      mask init:
      | [x y xp yp highstr lowstr maxy miny]=aeroimage('sixdofbody');
      | ports=aeroicon('aeroblk6dofbody','icon');
      mask Help: web(asbhelp('customvariablemass6dofquaternion'));
      mask StyleString: popup(Metric (MKS)|English (Velocity in ft/s)|English (Velocity in kts)),popup(Fixed|Simple Variable|Custom Variable),popup(Euler Angles|Quaternion),edit,edit,edit,edit,edit,edit,edit,edit,edit,edit,edit
      mask CallbackString: aeroicon('aeroblk6dofbody');|aeroicon('aeroblk6dofbody');|aeroicon('aeroblk6dofbody');|||||||||||
      mask Display:
      | port_label(ports(1).type,ports(1).port,ports(1).txt,'texmode','on');
      | port_label(ports(2).type,ports(2).port,ports(2).txt,'texmode','on');
      | port_label(ports(3).type,ports(3).port,ports(3).txt,'texmode','on');
      | port_label(ports(4).type,ports(4).port,ports(4).txt,'texmode','on');
      | port_label(ports(5).type,ports(5).port,ports(5).txt,'texmode','on');
      | port_label(ports(6).type,ports(6).port,ports(6).txt,'texmode','on');
      | port_label(ports(7).type,ports(7).port,ports(7).txt,'texmode','on');
      | port_label(ports(8).type,ports(8).port,ports(8).txt,'texmode','on');
      | port_label(ports(9).type,ports(9).port,ports(9).txt,'texmode','on');
      | port_label(ports(10).type,ports(10).port,ports(10).txt,'texmode','on');
      | port_label(ports(11).type,ports(11).port,ports(11).txt,'texmode','on');
      | port_label(ports(12).type,ports(12).port,ports(12).txt,'texmode','on');
      | port_label(ports(13).type,ports(13).port,ports(13).txt,'texmode','on');
      | port_label(ports(14).type,ports(14).port,ports(14).txt,'texmode','on');
      | port_label(ports(15).type,ports(15).port,ports(15).txt,'texmode','on');
      | port_label('output',9,'q_{ECI}','texmode','on');
      | port_label('output',10,'q_{ECI}_{0}','texmode','on');
      | text(0.5,maxy+0.05,highstr{:},'horizontalAlignment','center')
      | text(0.5,miny-0.05,lowstr{:},'horizontalAlignment','center')
      | plot(x,y);
      | patch(xp, yp);
  Display{13,15,22..23} (4 alike) : Display
  ECI to LLA : Subsystem
  Earth Gravity Model : Subsystem
  Ground : Ground
  Ground1 : Ground
  H-1 Engine Cluster : Subsystem
  Math Function : Math  Operator=square  SaturateOnIntegerOverflow=on
  Math Function1 : Math  Operator=sqrt  SaturateOnIntegerOverflow=on
  Product : Product  Multiplication=Matrix(*)  RndMeth=Zero
  Product1 : Product  RndMeth=Zero
  Relative Wind : Subsystem
  Retrorocket Motors : Subsystem
  Sum of Elements : Sum  Inputs=+  OutScaling=2^-10
  Terminator{1..8} (8 alike) : Terminator
  Vehicle Mass Properties : Subsystem
  airspeed (mps) : Display
  "alpha, ..." : Scope  NumInputPorts=2
      settings: TimeRange=150  YMin=97.45~-0.26  YMax=97.875~-0.247  SaveName=ScopeData5  Decimation=10
  height (m) : Display
  "qbar, mach" : Scope  NumInputPorts=3
      settings: TimeRange=150  YMin=3.9~6.77~0  YMax=5.4~6.795~17  Decimation=10
  lat_deg : Outport
  lon_deg : Outport  Port=2
  h_m : Outport  Port=3
  Xe_m : Outport  Port=4
  Ve_mps : Outport  Port=5
  alpha_deg : Outport  Port=6
  Vb_mps : Outport  Port=7
  q_ECI : Outport  Port=8
  omega_b_rps : Outport  Port=9  InitialOutput=[0.0 0.0 0.0]
  Ab_mps2 : Outport  Port=10  InitialOutput=[0.0 0.0 0.0]
  bPropellant_sensor_dry : Outport  Port=11
  B_b : Outport  Port=12
  CG_m : Outport  Port=13
  Vb_vec_mps : Outport  Port=14
  wires:
  COESA Atmosphere Model/4 -> Aerodynamic Forces and Moments/2(rho)
  Custom Variable Mass 6DoF (Quaternion)/2(Xe) -> ECI to LLA/2(ECI_pos (m)), [Xe_m], Relative Wind/1(Xe_m)
  ECI to LLA/3(h_ellp_m) -> COESA Atmosphere Model/1, h_m/1, height (m)/1, "Alt, V_ECI"/1
  Custom Variable Mass 6DoF (Quaternion)/4(DCM) -> [B_b], Relative Wind/2(B_b)
  [B_b] -> Product/1
  Earth Gravity Model/1(g (m/s^2)) -> Product/2
  Product/1 -> Product1/1, [g_b_mps2]
  Product1/1 -> Add/1
  Add/1 -> Custom Variable Mass 6DoF (Quaternion)/1(Forces)
  Vehicle Mass Properties/2(Cg_m) -> [Cg_m], CG_m/1
  Vehicle Mass Properties/3(I) -> Custom Variable Mass 6DoF (Quaternion)/6(I)
  COESA Atmosphere Model/2 -> Aerodynamic Forces and Moments/1(a_mps)
  Relative Wind/1(alpha_rad) -> Aerodynamic Forces and Moments/3(alpha_rad), Angle Conversion10/1
  Relative Wind/2(beta_rad) -> Angle Conversion9/1, Aerodynamic Forces and Moments/4(beta_rad)
  Relative Wind/3(V_mps) -> airspeed (mps)/1, Vb_mps/1, Aerodynamic Forces and Moments/5(V_mps)
  [Cg_m] -> Aerodynamic Forces and Moments/6(CG_m)
  Aerodynamic Forces and Moments/2(F_aero_N) -> [F_Aero_N]
  Aerodynamic Forces and Moments/3(M_aero_Nm) -> [M_Aero_Nm]
  [Xe_m] -> Earth Gravity Model/1(ECI_pos (m))
  Custom Variable Mass 6DoF (Quaternion)/8(Ab) -> Add2/1
  Custom Variable Mass 6DoF (Quaternion)/6(p,q,r) -> omega_b_rps/1
  Custom Variable Mass 6DoF (Quaternion)/7(pdot,qdot,rdot) -> Terminator1/1
  Custom Variable Mass 6DoF (Quaternion)/3(Euler) -> Terminator2/1
  Custom Variable Mass 6DoF (Quaternion)/9(q) -> [q_ECI]
  Custom Variable Mass 6DoF (Quaternion)/10(q0) -> Terminator3/1
  COESA Atmosphere Model/1 -> Terminator4/1
  COESA Atmosphere Model/3 -> Terminator5/1
  Aerodynamic Forces and Moments/4(qbar) -> Terminator6/1, "qbar, mach"/1
  Aerodynamic Forces and Moments/5(Mach) -> Terminator7/1, "qbar, mach"/2
  Ground/1 -> Custom Variable Mass 6DoF (Quaternion)/5(I_dot)
  Aerodynamic Forces and Moments/1(CP_m) -> Terminator8/1
  [Cg_m] -> H-1 Engine Cluster/2(CG_m)
  Angle Conversion4/1 -> lon_deg/1, Display13/1
  ECI to LLA/2(Lon_rad) -> Angle Conversion4/1
  ECI to LLA/1(Lat_rad) -> Angle Conversion5/1
  Angle Conversion5/1 -> Display15/1, lat_deg/1
  Ground1/1 -> Custom Variable Mass 6DoF (Quaternion)/3(m_dot)
  [F_engines_N] -> Add/3
  Custom Variable Mass 6DoF (Quaternion)/5(Vb) -> Relative Wind/3(Vb_mps), Vb_vec_mps/1
  Angle Conversion9/1 -> Display22/1, "alpha, ..."/2
  Angle Conversion10/1 -> Display23/1, "alpha, ..."/1, alpha_deg/1
  Vehicle Mass Properties/1(m_kg) -> Custom Variable Mass 6DoF (Quaternion)/4(mass), Product1/2
  [mdot_kg_sec] -> Vehicle Mass Properties/1(mdot_kg_per_sec)
  [M_engines_Nm] -> Add1/1
  Add1/1 -> Custom Variable Mass 6DoF (Quaternion)/2(Moments)
  [F_Aero_N] -> Add/2
  [M_Aero_Nm] -> Add1/2
  Add2/1 -> Ab_mps2/1, "qbar, mach"/3
  [g_b_mps2] -> Add2/2
  Custom Variable Mass 6DoF (Quaternion)/1(Ve) -> [Ve_mps], Math Function/1
  [Xe_m] -> Xe_m/1
  [Ve_mps] -> Ve_mps/1
  theta_GMST_rad/1 -> Earth Gravity Model/2(theta_GMST_rad), ECI to LLA/1(theta_GMST_rad)
  q_ECI_0/1 -> Custom Variable Mass 6DoF (Quaternion)/7(initial quaternion)
  Xe_0_m/1 -> Custom Variable Mass 6DoF (Quaternion)/8(Xe_initial_m)
  Vb_0_m/1 -> Custom Variable Mass 6DoF (Quaternion)/9(Vb_0_mps)
  T1_sec/1 -> H-1 Engine Cluster/1(T0_sec)
  bIECO/1 -> H-1 Engine Cluster/6(bIECO)
  bOECO/1 -> H-1 Engine Cluster/7(bOECO)
  H-1 Engine Cluster/3(mdot_kg_per_sec) -> [mdot_kg_sec]
  bEngineStart/1 -> H-1 Engine Cluster/8(bEngineStart)
  [q_ECI] -> q_ECI/1
  Vehicle Mass Properties/4(bPropellant_Sensor_dry) -> bPropellant_sensor_dry/1
  Math Function/1 -> Sum of Elements/1
  Sum of Elements/1 -> Math Function1/1
  Math Function1/1 -> "Alt, V_ECI"/2
  [B_b] -> B_b/1
  bStageSep/1 -> Retrorocket Motors/1(bRetroMotorStart), [bStageSep], Vehicle Mass Properties/2(bStageSep)
  Add3/1 -> [F_engines_N]
  Add4/1 -> [M_engines_Nm]
  Retrorocket Motors/2(Mb_N) -> Add4/2
  H-1 Engine Cluster/1(Fb_N) -> Add3/1
  H-1 Engine Cluster/2(Mb_Nm) -> Add4/1
  Retrorocket Motors/1(Fb_N) -> Add3/2
  [bStageSep] -> Aerodynamic Forces and Moments/7(bStageSep)
  beta_Y_deg/1 -> H-1 Engine Cluster/5(beta_Y_deg)
  beta_P_deg/1 -> H-1 Engine Cluster/4(beta_P_deg)
  beta_R_deg/1 -> H-1 Engine Cluster/3(beta_R_deg)

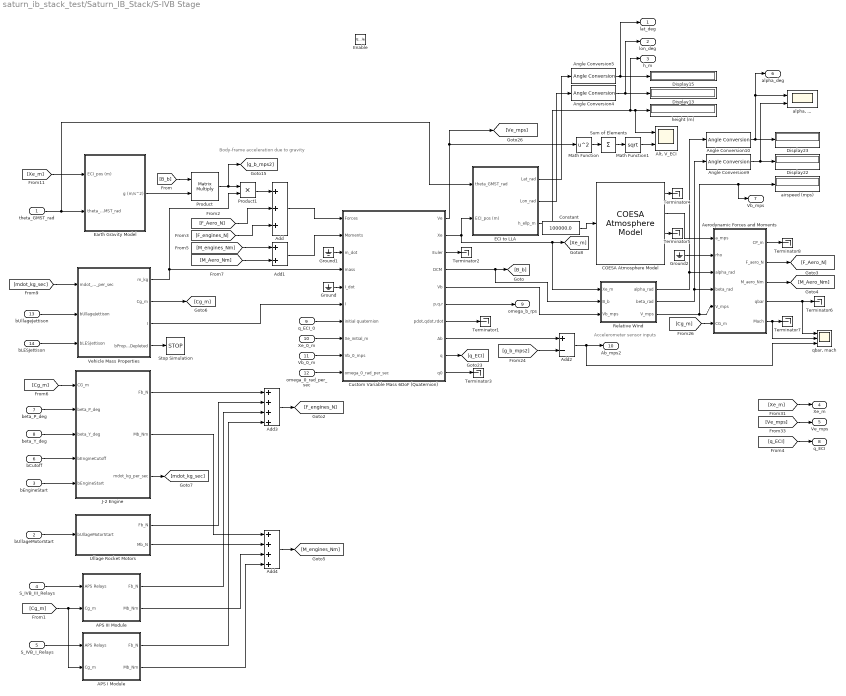
== system saturn_ib_stack_test/Saturn_IB_Stack/S-IVB Stage ==
  note: Accelerometer sensor inputs
  note: Body-frame acceleration
      | due to gravity
  theta_GMST_rad : Inport  Port=1  LatchInput=off
  bUllageMotorStart : Inport  Port=2  LatchInput=off
  bEngineStart : Inport  Port=3  LatchInput=off
  S_IVB_III_Relays : Inport  Port=4  LatchInput=off
  S_IVB_I_Relays : Inport  Port=5  LatchInput=off
  bCutoff : Inport  Port=6  LatchInput=off
  beta_P_deg : Inport  Port=7  LatchInput=off
  beta_Y_deg : Inport  Port=8  LatchInput=off
  q_ECI_0 : Inport  Port=9  LatchInput=off
  Xe_0_m : Inport  Port=10  LatchInput=off
  Vb_0_m : Inport  Port=11  LatchInput=off
  omega_0_rad_per_sec : Inport  Port=12  LatchInput=off
  bUllageJettison : Inport  Port=13  LatchInput=off
  bLESJettison : Inport  Port=14  LatchInput=off
  Enable : EnablePort
  APS I Module : Subsystem
  APS III Module : Subsystem
  Add : Sum  Inputs=+++  OutScaling=2^-10
  Add1 : Sum  OutScaling=2^-10
  Add2 : Sum  Inputs=+-  OutScaling=2^-10
  Add3 : Sum  Inputs=++++  OutScaling=2^-10
  Add4 : Sum  Inputs=++++  OutScaling=2^-10
  Aerodynamic Forces and Moments : Subsystem
  "Alt, V_ECI" : Scope  NumInputPorts=2
      settings: TimeRange=300  YMin=180000~3000  YMax=205000~8000  Decimation=10
  Angle Conversion{4..5,9..10} (4 alike) : aerolibconvert/Angle Conversion  IU=rad  OU=deg
  COESA Atmosphere Model : aerolibatmos2/COESA Atmosphere Model  units=Metric (MKS)  spec=1976 COESA-extended U.S. Standard Atmosphere  model=Profile  profile_var=High temperature  profile_percent=1%  profile_alt=5 km (16404 ft)  envelope_var=High temperature  envelope_percent=1%  action=Warning
  Constant : Constant  Value=100000.0
  Custom Variable Mass 6DoF (Quaternion) : Subsystem  mask(6DoF EoM (Body Axis)){units=Metric (MKS), mtype=Custom Variable, rep=Quaternion, xme_0=[0 0 0], Vm_0=[0 0 0], eul_0=[0 0 0], pm_0=[0 0 0], mass_0=1.0, mass_e=0, mass_f=0, inertia=eye(3), inertia_e=eye(3), inertia_f=eye(3), k_quat=1.0}
      mask prompts: mtype "Mass type:"; rep "Representation:"; xme_0 "Initial position in inertial axes [Xe,Ye,Ze]:"; Vm_0 "Initial velocity in body axes [U,v,w]:"; eul_0 "Initial Euler orientation [roll, pitch, yaw]:"; pm_0 "Initial body rotation rates [p,q,r]:"; mass_0 "Initial mass:"; mass_e "Empty mass:"; mass_f "Full mass:"; inertia_e "Empty inertia matrix:"; inertia_f "Full inertia matrix:"; k_quat "Gain for quaternion normalization:"
      mask help: Integrate the six-degrees-of-freedom equations of motion using an Euler angle representation for the orientation of the body in space.
      mask init:
      | [x y xp yp highstr lowstr maxy miny]=aeroimage('sixdofbody');
      | ports=aeroicon('aeroblk6dofbody','icon');
      mask Help: web(asbhelp('customvariablemass6dofquaternion'));
      mask StyleString: popup(Metric (MKS)|English (Velocity in ft/s)|English (Velocity in kts)),popup(Fixed|Simple Variable|Custom Variable),popup(Euler Angles|Quaternion),edit,edit,edit,edit,edit,edit,edit,edit,edit,edit,edit
      mask CallbackString: aeroicon('aeroblk6dofbody');|aeroicon('aeroblk6dofbody');|aeroicon('aeroblk6dofbody');|||||||||||
      mask Display:
      | port_label(ports(1).type,ports(1).port,ports(1).txt,'texmode','on');
      | port_label(ports(2).type,ports(2).port,ports(2).txt,'texmode','on');
      | port_label(ports(3).type,ports(3).port,ports(3).txt,'texmode','on');
      | port_label(ports(4).type,ports(4).port,ports(4).txt,'texmode','on');
      | port_label(ports(5).type,ports(5).port,ports(5).txt,'texmode','on');
      | port_label(ports(6).type,ports(6).port,ports(6).txt,'texmode','on');
      | port_label(ports(7).type,ports(7).port,ports(7).txt,'texmode','on');
      | port_label(ports(8).type,ports(8).port,ports(8).txt,'texmode','on');
      | port_label(ports(9).type,ports(9).port,ports(9).txt,'texmode','on');
      | port_label(ports(10).type,ports(10).port,ports(10).txt,'texmode','on');
      | port_label(ports(11).type,ports(11).port,ports(11).txt,'texmode','on');
      | port_label(ports(12).type,ports(12).port,ports(12).txt,'texmode','on');
      | port_label(ports(13).type,ports(13).port,ports(13).txt,'texmode','on');
      | port_label(ports(14).type,ports(14).port,ports(14).txt,'texmode','on');
      | port_label(ports(15).type,ports(15).port,ports(15).txt,'texmode','on');
      | port_label('output',9,'q_{ECI}','texmode','on');
      | port_label('output',10,'q_{ECI}_{0}','texmode','on');
      | text(0.5,maxy+0.05,highstr{:},'horizontalAlignment','center')
      | text(0.5,miny-0.05,lowstr{:},'horizontalAlignment','center')
      | plot(x,y);
      | patch(xp, yp);
  Display{13,15,22..23} (4 alike) : Display
  ECI to LLA : Subsystem
  Earth Gravity Model : Subsystem
  Ground : Ground
  Ground1 : Ground
  Ground2 : Ground
  J-2 Engine : Subsystem
  Math Function : Math  Operator=square  SaturateOnIntegerOverflow=on
  Math Function1 : Math  Operator=sqrt  SaturateOnIntegerOverflow=on
  Product : Product  Multiplication=Matrix(*)  RndMeth=Zero
  Product1 : Product  RndMeth=Zero
  Relative Wind : Subsystem
  Stop Simulation : Stop
  Sum of Elements : Sum  Inputs=+  OutScaling=2^-10
  Terminator{1..8} (8 alike) : Terminator
  Ullage Rocket Motors : Subsystem
  Vehicle Mass Properties : Subsystem
  airspeed (mps) : Display
  "alpha, ..." : Scope  NumInputPorts=2
      settings: TimeRange=150  YMin=24.05~-0.464  YMax=24.55~-0.449  SaveName=ScopeData5  Decimation=10
  height (m) : Display
  "qbar, mach" : Scope  NumInputPorts=3
      settings: TimeRange=140  YMin=-1~8.0125~0  YMax=1~8.05~8  Decimation=10
  lat_deg : Outport
  lon_deg : Outport  Port=2
  h_m : Outport  Port=3
  Xe_m : Outport  Port=4
  Ve_mps : Outport  Port=5
  alpha_deg : Outport  Port=6
  Vb_mps : Outport  Port=7
  q_ECI : Outport  Port=8  InitialOutput=[1.0 0.0 0.0 0.0]
  omega_b_rps : Outport  Port=9  OutputWhenDisabled=reset  InitialOutput=[0.0 0.0 0.0]
  Ab_mps2 : Outport  Port=10  InitialOutput=[0.001 0.00 0.00]
  wires:
  Custom Variable Mass 6DoF (Quaternion)/2(Xe) -> ECI to LLA/2(ECI_pos (m)), [Xe_m], Relative Wind/1(Xe_m)
  ECI to LLA/3(h_ellp_m) -> h_m/1, height (m)/1, "Alt, V_ECI"/1
  Custom Variable Mass 6DoF (Quaternion)/4(DCM) -> [B_b], Relative Wind/2(B_b)
  [B_b] -> Product/1
  Earth Gravity Model/1(g (m/s^2)) -> Product/2
  Product/1 -> Product1/1, [g_b_mps2]
  Product1/1 -> Add/1
  Add/1 -> Custom Variable Mass 6DoF (Quaternion)/1(Forces)
  Vehicle Mass Properties/2(Cg_m) -> [Cg_m]
  Vehicle Mass Properties/3(I) -> Custom Variable Mass 6DoF (Quaternion)/6(I)
  COESA Atmosphere Model/2 -> Aerodynamic Forces and Moments/1(a_mps)
  Relative Wind/1(alpha_rad) -> Aerodynamic Forces and Moments/3(alpha_rad), Angle Conversion10/1
  Relative Wind/2(beta_rad) -> Angle Conversion9/1, Aerodynamic Forces and Moments/4(beta_rad)
  Relative Wind/3(V_mps) -> Aerodynamic Forces and Moments/5(V_mps), airspeed (mps)/1, Vb_mps/1
  [Cg_m] -> Aerodynamic Forces and Moments/6(CG_m)
  Aerodynamic Forces and Moments/2(F_aero_N) -> [F_Aero_N]
  Aerodynamic Forces and Moments/3(M_aero_Nm) -> [M_Aero_Nm]
  [Xe_m] -> Earth Gravity Model/1(ECI_pos (m))
  J-2 Engine/1(Fb_N) -> Add3/1
  Custom Variable Mass 6DoF (Quaternion)/8(Ab) -> Add2/1
  Custom Variable Mass 6DoF (Quaternion)/6(p,q,r) -> omega_b_rps/1
  Custom Variable Mass 6DoF (Quaternion)/7(pdot,qdot,rdot) -> Terminator1/1
  Custom Variable Mass 6DoF (Quaternion)/3(Euler) -> Terminator2/1
  Custom Variable Mass 6DoF (Quaternion)/9(q) -> [q_ECI]
  Custom Variable Mass 6DoF (Quaternion)/10(q0) -> Terminator3/1
  COESA Atmosphere Model/1 -> Terminator4/1
  COESA Atmosphere Model/3 -> Terminator5/1
  Aerodynamic Forces and Moments/4(qbar) -> Terminator6/1, "qbar, mach"/1
  Aerodynamic Forces and Moments/5(Mach) -> Terminator7/1, "qbar, mach"/2
  Ground/1 -> Custom Variable Mass 6DoF (Quaternion)/5(I_dot)
  Aerodynamic Forces and Moments/1(CP_m) -> Terminator8/1
  [Cg_m] -> J-2 Engine/1(CG_m)
  Angle Conversion4/1 -> lon_deg/1, Display13/1
  ECI to LLA/2(Lon_rad) -> Angle Conversion4/1
  ECI to LLA/1(Lat_rad) -> Angle Conversion5/1
  Angle Conversion5/1 -> Display15/1, lat_deg/1
  Ground1/1 -> Custom Variable Mass 6DoF (Quaternion)/3(m_dot)
  [F_engines_N] -> Add/3
  Custom Variable Mass 6DoF (Quaternion)/5(Vb) -> Relative Wind/3(Vb_mps)
  Angle Conversion9/1 -> Display22/1, "alpha, ..."/2
  Angle Conversion10/1 -> Display23/1, "alpha, ..."/1, alpha_deg/1
  Vehicle Mass Properties/1(m_kg) -> Custom Variable Mass 6DoF (Quaternion)/4(mass), Product1/2
  [mdot_kg_sec] -> Vehicle Mass Properties/1(mdot_kg_per_sec)
  J-2 Engine/2(Mb_Nm) -> Add4/1
  Add1/1 -> Custom Variable Mass 6DoF (Quaternion)/2(Moments)
  Add2/1 -> Ab_mps2/1, "qbar, mach"/3
  [g_b_mps2] -> Add2/2
  Custom Variable Mass 6DoF (Quaternion)/1(Ve) -> [Ve_mps], Math Function/1
  [Xe_m] -> Xe_m/1
  [Ve_mps] -> Ve_mps/1
  theta_GMST_rad/1 -> Earth Gravity Model/2(theta_GMST_rad), ECI to LLA/1(theta_GMST_rad)
  q_ECI_0/1 -> Custom Variable Mass 6DoF (Quaternion)/7(initial quaternion)
  Xe_0_m/1 -> Custom Variable Mass 6DoF (Quaternion)/8(Xe_initial_m)
  Vb_0_m/1 -> Custom Variable Mass 6DoF (Quaternion)/9(Vb_0_mps)
  beta_P_deg/1 -> J-2 Engine/2(beta_P_deg)
  beta_Y_deg/1 -> J-2 Engine/3(beta_Y_deg)
  bCutoff/1 -> J-2 Engine/4(bEngineCutoff)
  J-2 Engine/3(mdot_kg_per_sec) -> [mdot_kg_sec]
  bEngineStart/1 -> J-2 Engine/5(bEngineStart)
  [q_ECI] -> q_ECI/1
  Math Function/1 -> Sum of Elements/1
  Sum of Elements/1 -> Math Function1/1
  Math Function1/1 -> "Alt, V_ECI"/2
  omega_0_rad_per_sec/1 -> Custom Variable Mass 6DoF (Quaternion)/10(omega_0_rad_per_sec)
  Add3/1 -> [F_engines_N]
  Add4/1 -> [M_engines_Nm]
  bUllageMotorStart/1 -> Ullage Rocket Motors/1(bUllageMotorStart)
  S_IVB_III_Relays/1 -> APS III Module/1(APS Relays)
  S_IVB_I_Relays/1 -> APS I Module/1(APS Relays)
  [M_engines_Nm] -> Add1/1
  Ullage Rocket Motors/1(Fb_N) -> Add3/2
  Ullage Rocket Motors/2(Mb_N) -> Add4/2
  [Cg_m] -> APS III Module/2(Cg_m), APS I Module/2(Cg_m)
  APS III Module/1(Fb_N) -> Add3/3
  APS III Module/2(Mb_Nm) -> Add4/3
  APS I Module/1(Fb_N) -> Add3/4
  APS I Module/2(Mb_Nm) -> Add4/4
  Ground2/1 -> Aerodynamic Forces and Moments/2(rho)
  Constant/1 -> COESA Atmosphere Model/1
  [F_Aero_N] -> Add/2
  [M_Aero_Nm] -> Add1/2
  Vehicle Mass Properties/4(bPropellantDepleted) -> Stop Simulation/1
  bUllageJettison/1 -> Vehicle Mass Properties/2(bUllageJettison)
  bLESJettison/1 -> Vehicle Mass Properties/3(bLESJettison)
